simulink model "Thirtybussys1"  (R2021a)
settings: Solver=VariableStepAuto  StartTime=0.0  StopTime=4.0  RelTol=1e-3
libraries: spsFourierLib x60, spsThreePhaseSeriesRLCBranchLib x41, spsThreePhaseVIMeasurementLib x30, spsThreePhaseSeriesRLCLoadLib x21, spsThreePhaseSourceLib x6, spsThreePhaseTransformerTwoWindingsLib x6, spsThreePhaseFaultLib x2, spspowerguiLib x1
(part 2 of 2)

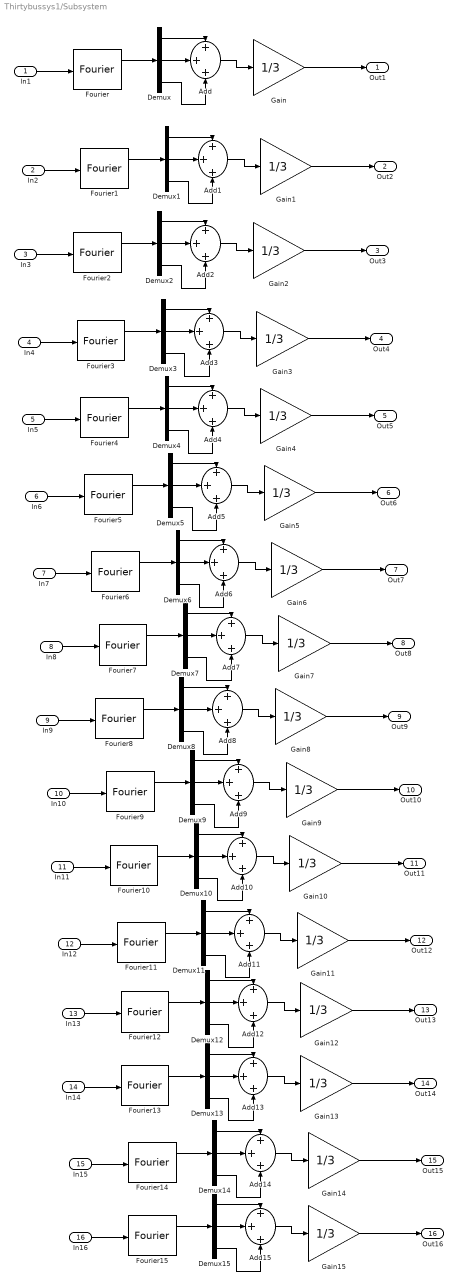
== system Thirtybussys1/Subsystem ==
  In1 : Inport
  In2 : Inport  Port=2
  In3 : Inport  Port=3
  In4 : Inport  Port=4
  In5 : Inport  Port=5
  In6 : Inport  Port=6
  In7 : Inport  Port=7
  In8 : Inport  Port=8
  In9 : Inport  Port=9
  In10 : Inport  Port=10
  In11 : Inport  Port=11
  In12 : Inport  Port=12
  In13 : Inport  Port=13
  In14 : Inport  Port=14
  In15 : Inport  Port=15
  In16 : Inport  Port=16
  Add{,1..15} (16 alike) : Sum  Inputs=+++
  Demux{,1..15} (16 alike) : Demux  Outputs=3
  Fourier{,1..15} (16 alike) : spsFourierLib/Fourier  Freq=60  n=1  InInit=[0, 0]  Ts=50e-6
      settings: SourceProductBaseCode=PS
  Gain{,1..15} (16 alike) : Gain  Gain=1/3
  Out1 : Outport
  Out2 : Outport  Port=2
  Out3 : Outport  Port=3
  Out4 : Outport  Port=4
  Out5 : Outport  Port=5
  Out6 : Outport  Port=6
  Out7 : Outport  Port=7
  Out8 : Outport  Port=8
  Out9 : Outport  Port=9
  Out10 : Outport  Port=10
  Out11 : Outport  Port=11
  Out12 : Outport  Port=12
  Out13 : Outport  Port=13
  Out14 : Outport  Port=14
  Out15 : Outport  Port=15
  Out16 : Outport  Port=16
  wires:
  In1/1 -> Fourier/1
  Add/1 -> Gain/1
  Gain/1 -> Out1/1
  Fourier/1 -> Demux/1
  Demux/1 -> Add/1
  Demux/2 -> Add/2
  Demux/3 -> Add/3
  Demux1/3 -> Add1/3
  Demux1/2 -> Add1/2
  In2/1 -> Fourier1/1
  Fourier1/1 -> Demux1/1
  Demux1/1 -> Add1/1
  Add1/1 -> Gain1/1
  Gain1/1 -> Out2/1
  Demux2/3 -> Add2/3
  Demux2/2 -> Add2/2
  In3/1 -> Fourier2/1
  Fourier2/1 -> Demux2/1
  Demux2/1 -> Add2/1
  Add2/1 -> Gain2/1
  Gain2/1 -> Out3/1
  Demux3/3 -> Add3/3
  Demux3/2 -> Add3/2
  In4/1 -> Fourier3/1
  Fourier3/1 -> Demux3/1
  Demux3/1 -> Add3/1
  Add3/1 -> Gain3/1
  Gain3/1 -> Out4/1
  Demux4/3 -> Add4/3
  Demux4/2 -> Add4/2
  In5/1 -> Fourier4/1
  Fourier4/1 -> Demux4/1
  Demux4/1 -> Add4/1
  Add4/1 -> Gain4/1
  Gain4/1 -> Out5/1
  Demux5/3 -> Add5/3
  Demux5/2 -> Add5/2
  In6/1 -> Fourier5/1
  Fourier5/1 -> Demux5/1
  Demux5/1 -> Add5/1
  Add5/1 -> Gain5/1
  Gain5/1 -> Out6/1
  Demux6/3 -> Add6/3
  Demux6/2 -> Add6/2
  In7/1 -> Fourier6/1
  Fourier6/1 -> Demux6/1
  Demux6/1 -> Add6/1
  Add6/1 -> Gain6/1
  Gain6/1 -> Out7/1
  Demux7/3 -> Add7/3
  Demux7/2 -> Add7/2
  In8/1 -> Fourier7/1
  Fourier7/1 -> Demux7/1
  Demux7/1 -> Add7/1
  Add7/1 -> Gain7/1
  Gain7/1 -> Out8/1
  Demux8/3 -> Add8/3
  Demux8/2 -> Add8/2
  In9/1 -> Fourier8/1
  Fourier8/1 -> Demux8/1
  Demux8/1 -> Add8/1
  Add8/1 -> Gain8/1
  Gain8/1 -> Out9/1
  Demux9/3 -> Add9/3
  Demux9/2 -> Add9/2
  In10/1 -> Fourier9/1
  Fourier9/1 -> Demux9/1
  Demux9/1 -> Add9/1
  Add9/1 -> Gain9/1
  Gain9/1 -> Out10/1
  Demux10/3 -> Add10/3
  Demux10/2 -> Add10/2
  In11/1 -> Fourier10/1
  Fourier10/1 -> Demux10/1
  Demux10/1 -> Add10/1
  Add10/1 -> Gain10/1
  Gain10/1 -> Out11/1
  Demux11/3 -> Add11/3
  Demux11/2 -> Add11/2
  In12/1 -> Fourier11/1
  Fourier11/1 -> Demux11/1
  Demux11/1 -> Add11/1
  Add11/1 -> Gain11/1
  Gain11/1 -> Out12/1
  Demux12/3 -> Add12/3
  Demux12/2 -> Add12/2
  In13/1 -> Fourier12/1
  Fourier12/1 -> Demux12/1
  Demux12/1 -> Add12/1
  Add12/1 -> Gain12/1
  Gain12/1 -> Out13/1
  Demux13/3 -> Add13/3
  Demux13/2 -> Add13/2
  In14/1 -> Fourier13/1
  Fourier13/1 -> Demux13/1
  Demux13/1 -> Add13/1
  Add13/1 -> Gain13/1
  Gain13/1 -> Out14/1
  Demux14/3 -> Add14/3
  Demux14/2 -> Add14/2
  In15/1 -> Fourier14/1
  Fourier14/1 -> Demux14/1
  Demux14/1 -> Add14/1
  Add14/1 -> Gain14/1
  Gain14/1 -> Out15/1
  Demux15/2 -> Add15/2
  Fourier15/1 -> Demux15/1
  Gain15/1 -> Out16/1
  In16/1 -> Fourier15/1
  Demux15/3 -> Add15/3
  Add15/1 -> Gain15/1
  Demux15/1 -> Add15/1

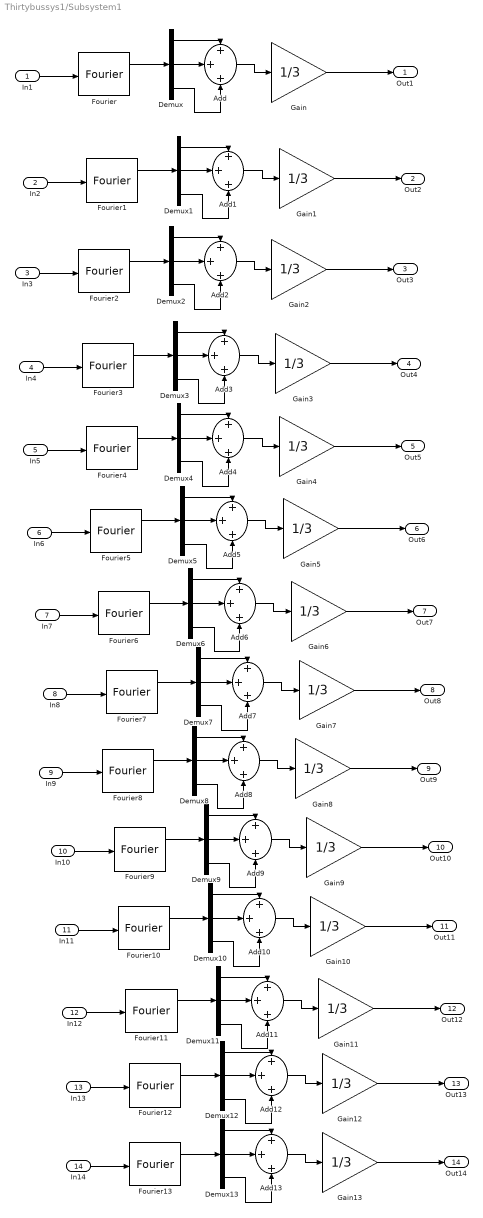
== system Thirtybussys1/Subsystem1 ==
  In1 : Inport
  In2 : Inport  Port=2
  In3 : Inport  Port=3
  In4 : Inport  Port=4
  In5 : Inport  Port=5
  In6 : Inport  Port=6
  In7 : Inport  Port=7
  In8 : Inport  Port=8
  In9 : Inport  Port=9
  In10 : Inport  Port=10
  In11 : Inport  Port=11
  In12 : Inport  Port=12
  In13 : Inport  Port=13
  In14 : Inport  Port=14
  Add{,1..13} (14 alike) : Sum  Inputs=+++
  Demux{,1..13} (14 alike) : Demux  Outputs=3
  Fourier{,1..13} (14 alike) : spsFourierLib/Fourier  Freq=60  n=1  InInit=[0, 0]  Ts=50e-6
      settings: SourceProductBaseCode=PS
  Gain{,1..13} (14 alike) : Gain  Gain=1/3
  Out1 : Outport
  Out2 : Outport  Port=2
  Out3 : Outport  Port=3
  Out4 : Outport  Port=4
  Out5 : Outport  Port=5
  Out6 : Outport  Port=6
  Out7 : Outport  Port=7
  Out8 : Outport  Port=8
  Out9 : Outport  Port=9
  Out10 : Outport  Port=10
  Out11 : Outport  Port=11
  Out12 : Outport  Port=12
  Out13 : Outport  Port=13
  Out14 : Outport  Port=14
  wires:
  In1/1 -> Fourier/1
  Add/1 -> Gain/1
  Gain/1 -> Out1/1
  Fourier/1 -> Demux/1
  Demux/1 -> Add/1
  Demux/2 -> Add/2
  Demux/3 -> Add/3
  Demux1/3 -> Add1/3
  Demux1/2 -> Add1/2
  In2/1 -> Fourier1/1
  Fourier1/1 -> Demux1/1
  Demux1/1 -> Add1/1
  Add1/1 -> Gain1/1
  Gain1/1 -> Out2/1
  Demux2/3 -> Add2/3
  Demux2/2 -> Add2/2
  In3/1 -> Fourier2/1
  Fourier2/1 -> Demux2/1
  Demux2/1 -> Add2/1
  Add2/1 -> Gain2/1
  Gain2/1 -> Out3/1
  Demux3/3 -> Add3/3
  Demux3/2 -> Add3/2
  In4/1 -> Fourier3/1
  Fourier3/1 -> Demux3/1
  Demux3/1 -> Add3/1
  Add3/1 -> Gain3/1
  Gain3/1 -> Out4/1
  Demux4/3 -> Add4/3
  Demux4/2 -> Add4/2
  In5/1 -> Fourier4/1
  Fourier4/1 -> Demux4/1
  Demux4/1 -> Add4/1
  Add4/1 -> Gain4/1
  Gain4/1 -> Out5/1
  Demux5/3 -> Add5/3
  Demux5/2 -> Add5/2
  In6/1 -> Fourier5/1
  Fourier5/1 -> Demux5/1
  Demux5/1 -> Add5/1
  Add5/1 -> Gain5/1
  Gain5/1 -> Out6/1
  Demux6/3 -> Add6/3
  Demux6/2 -> Add6/2
  In7/1 -> Fourier6/1
  Fourier6/1 -> Demux6/1
  Demux6/1 -> Add6/1
  Add6/1 -> Gain6/1
  Gain6/1 -> Out7/1
  Demux7/3 -> Add7/3
  Demux7/2 -> Add7/2
  In8/1 -> Fourier7/1
  Fourier7/1 -> Demux7/1
  Demux7/1 -> Add7/1
  Add7/1 -> Gain7/1
  Gain7/1 -> Out8/1
  Demux8/3 -> Add8/3
  Demux8/2 -> Add8/2
  In9/1 -> Fourier8/1
  Fourier8/1 -> Demux8/1
  Demux8/1 -> Add8/1
  Add8/1 -> Gain8/1
  Gain8/1 -> Out9/1
  Demux9/3 -> Add9/3
  Demux9/2 -> Add9/2
  In10/1 -> Fourier9/1
  Fourier9/1 -> Demux9/1
  Demux9/1 -> Add9/1
  Add9/1 -> Gain9/1
  Gain9/1 -> Out10/1
  Demux10/3 -> Add10/3
  Demux10/2 -> Add10/2
  In11/1 -> Fourier10/1
  Fourier10/1 -> Demux10/1
  Demux10/1 -> Add10/1
  Add10/1 -> Gain10/1
  Gain10/1 -> Out11/1
  Demux11/3 -> Add11/3
  Demux11/2 -> Add11/2
  In12/1 -> Fourier11/1
  Fourier11/1 -> Demux11/1
  Demux11/1 -> Add11/1
  Add11/1 -> Gain11/1
  Gain11/1 -> Out12/1
  Demux12/3 -> Add12/3
  Demux12/2 -> Add12/2
  In13/1 -> Fourier12/1
  Fourier12/1 -> Demux12/1
  Demux12/1 -> Add12/1
  Add12/1 -> Gain12/1
  Gain12/1 -> Out13/1
  Demux13/3 -> Add13/3
  Demux13/2 -> Add13/2
  In14/1 -> Fourier13/1
  Fourier13/1 -> Demux13/1
  Demux13/1 -> Add13/1
  Add13/1 -> Gain13/1
  Gain13/1 -> Out14/1

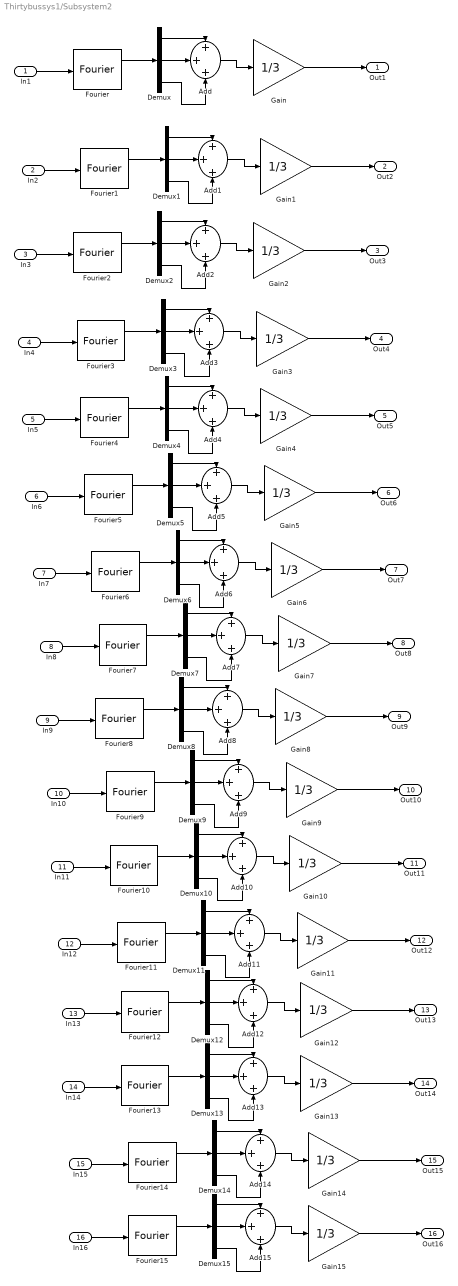
== system Thirtybussys1/Subsystem2 ==
  In1 : Inport
  In2 : Inport  Port=2
  In3 : Inport  Port=3
  In4 : Inport  Port=4
  In5 : Inport  Port=5
  In6 : Inport  Port=6
  In7 : Inport  Port=7
  In8 : Inport  Port=8
  In9 : Inport  Port=9
  In10 : Inport  Port=10
  In11 : Inport  Port=11
  In12 : Inport  Port=12
  In13 : Inport  Port=13
  In14 : Inport  Port=14
  In15 : Inport  Port=15
  In16 : Inport  Port=16
  Add{,1..15} (16 alike) : Sum  Inputs=+++
  Demux{,1..15} (16 alike) : Demux  Outputs=3
  Fourier{,1..15} (16 alike) : spsFourierLib/Fourier  Freq=60  n=1  InInit=[0, 0]  Ts=50e-6
      settings: SourceProductBaseCode=PS
  Gain{,1..15} (16 alike) : Gain  Gain=1/3
  Out1 : Outport
  Out2 : Outport  Port=2
  Out3 : Outport  Port=3
  Out4 : Outport  Port=4
  Out5 : Outport  Port=5
  Out6 : Outport  Port=6
  Out7 : Outport  Port=7
  Out8 : Outport  Port=8
  Out9 : Outport  Port=9
  Out10 : Outport  Port=10
  Out11 : Outport  Port=11
  Out12 : Outport  Port=12
  Out13 : Outport  Port=13
  Out14 : Outport  Port=14
  Out15 : Outport  Port=15
  Out16 : Outport  Port=16
  wires:
  In1/1 -> Fourier/1
  Add/1 -> Gain/1
  Gain/1 -> Out1/1
  Fourier/1 -> Demux/1
  Demux/1 -> Add/1
  Demux/2 -> Add/2
  Demux/3 -> Add/3
  Demux1/3 -> Add1/3
  Demux1/2 -> Add1/2
  In2/1 -> Fourier1/1
  Fourier1/1 -> Demux1/1
  Demux1/1 -> Add1/1
  Add1/1 -> Gain1/1
  Gain1/1 -> Out2/1
  Demux2/3 -> Add2/3
  Demux2/2 -> Add2/2
  In3/1 -> Fourier2/1
  Fourier2/1 -> Demux2/1
  Demux2/1 -> Add2/1
  Add2/1 -> Gain2/1
  Gain2/1 -> Out3/1
  Demux3/3 -> Add3/3
  Demux3/2 -> Add3/2
  In4/1 -> Fourier3/1
  Fourier3/1 -> Demux3/1
  Demux3/1 -> Add3/1
  Add3/1 -> Gain3/1
  Gain3/1 -> Out4/1
  Demux4/3 -> Add4/3
  Demux4/2 -> Add4/2
  In5/1 -> Fourier4/1
  Fourier4/1 -> Demux4/1
  Demux4/1 -> Add4/1
  Add4/1 -> Gain4/1
  Gain4/1 -> Out5/1
  Demux5/3 -> Add5/3
  Demux5/2 -> Add5/2
  In6/1 -> Fourier5/1
  Fourier5/1 -> Demux5/1
  Demux5/1 -> Add5/1
  Add5/1 -> Gain5/1
  Gain5/1 -> Out6/1
  Demux6/3 -> Add6/3
  Demux6/2 -> Add6/2
  In7/1 -> Fourier6/1
  Fourier6/1 -> Demux6/1
  Demux6/1 -> Add6/1
  Add6/1 -> Gain6/1
  Gain6/1 -> Out7/1
  Demux7/3 -> Add7/3
  Demux7/2 -> Add7/2
  In8/1 -> Fourier7/1
  Fourier7/1 -> Demux7/1
  Demux7/1 -> Add7/1
  Add7/1 -> Gain7/1
  Gain7/1 -> Out8/1
  Demux8/3 -> Add8/3
  Demux8/2 -> Add8/2
  In9/1 -> Fourier8/1
  Fourier8/1 -> Demux8/1
  Demux8/1 -> Add8/1
  Add8/1 -> Gain8/1
  Gain8/1 -> Out9/1
  Demux9/3 -> Add9/3
  Demux9/2 -> Add9/2
  In10/1 -> Fourier9/1
  Fourier9/1 -> Demux9/1
  Demux9/1 -> Add9/1
  Add9/1 -> Gain9/1
  Gain9/1 -> Out10/1
  Demux10/3 -> Add10/3
  Demux10/2 -> Add10/2
  In11/1 -> Fourier10/1
  Fourier10/1 -> Demux10/1
  Demux10/1 -> Add10/1
  Add10/1 -> Gain10/1
  Gain10/1 -> Out11/1
  Demux11/3 -> Add11/3
  Demux11/2 -> Add11/2
  In12/1 -> Fourier11/1
  Fourier11/1 -> Demux11/1
  Demux11/1 -> Add11/1
  Add11/1 -> Gain11/1
  Gain11/1 -> Out12/1
  Demux12/3 -> Add12/3
  Demux12/2 -> Add12/2
  In13/1 -> Fourier12/1
  Fourier12/1 -> Demux12/1
  Demux12/1 -> Add12/1
  Add12/1 -> Gain12/1
  Gain12/1 -> Out13/1
  Demux13/3 -> Add13/3
  Demux13/2 -> Add13/2
  In14/1 -> Fourier13/1
  Fourier13/1 -> Demux13/1
  Demux13/1 -> Add13/1
  Add13/1 -> Gain13/1
  Gain13/1 -> Out14/1
  Demux14/3 -> Add14/3
  Demux14/2 -> Add14/2
  In15/1 -> Fourier14/1
  Fourier14/1 -> Demux14/1
  Demux14/1 -> Add14/1
  Add14/1 -> Gain14/1
  Gain14/1 -> Out15/1
  Demux15/2 -> Add15/2
  Fourier15/1 -> Demux15/1
  Gain15/1 -> Out16/1
  In16/1 -> Fourier15/1
  Demux15/3 -> Add15/3
  Add15/1 -> Gain15/1
  Demux15/1 -> Add15/1

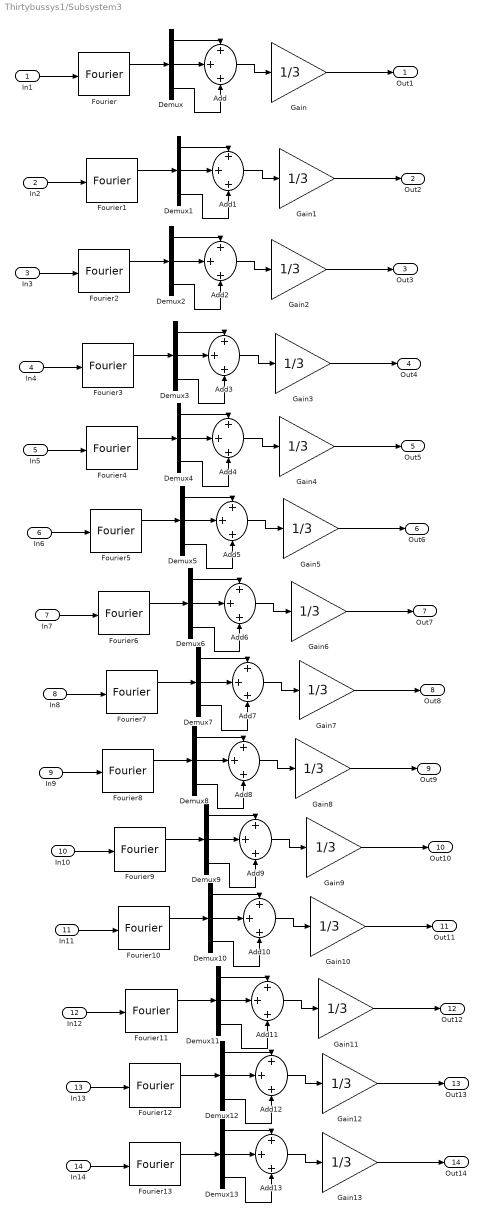
== system Thirtybussys1/Subsystem3 ==
  In1 : Inport
  In2 : Inport  Port=2
  In3 : Inport  Port=3
  In4 : Inport  Port=4
  In5 : Inport  Port=5
  In6 : Inport  Port=6
  In7 : Inport  Port=7
  In8 : Inport  Port=8
  In9 : Inport  Port=9
  In10 : Inport  Port=10
  In11 : Inport  Port=11
  In12 : Inport  Port=12
  In13 : Inport  Port=13
  In14 : Inport  Port=14
  Add{,1..13} (14 alike) : Sum  Inputs=+++
  Demux{,1..13} (14 alike) : Demux  Outputs=3
  Fourier{,1..13} (14 alike) : spsFourierLib/Fourier  Freq=60  n=1  InInit=[0, 0]  Ts=50e-6
      settings: SourceProductBaseCode=PS
  Gain{,1..13} (14 alike) : Gain  Gain=1/3
  Out1 : Outport
  Out2 : Outport  Port=2
  Out3 : Outport  Port=3
  Out4 : Outport  Port=4
  Out5 : Outport  Port=5
  Out6 : Outport  Port=6
  Out7 : Outport  Port=7
  Out8 : Outport  Port=8
  Out9 : Outport  Port=9
  Out10 : Outport  Port=10
  Out11 : Outport  Port=11
  Out12 : Outport  Port=12
  Out13 : Outport  Port=13
  Out14 : Outport  Port=14
  wires:
  In1/1 -> Fourier/1
  Add/1 -> Gain/1
  Gain/1 -> Out1/1
  Fourier/1 -> Demux/1
  Demux/1 -> Add/1
  Demux/2 -> Add/2
  Demux/3 -> Add/3
  Demux1/3 -> Add1/3
  Demux1/2 -> Add1/2
  In2/1 -> Fourier1/1
  Fourier1/1 -> Demux1/1
  Demux1/1 -> Add1/1
  Add1/1 -> Gain1/1
  Gain1/1 -> Out2/1
  Demux2/3 -> Add2/3
  Demux2/2 -> Add2/2
  In3/1 -> Fourier2/1
  Fourier2/1 -> Demux2/1
  Demux2/1 -> Add2/1
  Add2/1 -> Gain2/1
  Gain2/1 -> Out3/1
  Demux3/3 -> Add3/3
  Demux3/2 -> Add3/2
  In4/1 -> Fourier3/1
  Fourier3/1 -> Demux3/1
  Demux3/1 -> Add3/1
  Add3/1 -> Gain3/1
  Gain3/1 -> Out4/1
  Demux4/3 -> Add4/3
  Demux4/2 -> Add4/2
  In5/1 -> Fourier4/1
  Fourier4/1 -> Demux4/1
  Demux4/1 -> Add4/1
  Add4/1 -> Gain4/1
  Gain4/1 -> Out5/1
  Demux5/3 -> Add5/3
  Demux5/2 -> Add5/2
  In6/1 -> Fourier5/1
  Fourier5/1 -> Demux5/1
  Demux5/1 -> Add5/1
  Add5/1 -> Gain5/1
  Gain5/1 -> Out6/1
  Demux6/3 -> Add6/3
  Demux6/2 -> Add6/2
  In7/1 -> Fourier6/1
  Fourier6/1 -> Demux6/1
  Demux6/1 -> Add6/1
  Add6/1 -> Gain6/1
  Gain6/1 -> Out7/1
  Demux7/3 -> Add7/3
  Demux7/2 -> Add7/2
  In8/1 -> Fourier7/1
  Fourier7/1 -> Demux7/1
  Demux7/1 -> Add7/1
  Add7/1 -> Gain7/1
  Gain7/1 -> Out8/1
  Demux8/3 -> Add8/3
  Demux8/2 -> Add8/2
  In9/1 -> Fourier8/1
  Fourier8/1 -> Demux8/1
  Demux8/1 -> Add8/1
  Add8/1 -> Gain8/1
  Gain8/1 -> Out9/1
  Demux9/3 -> Add9/3
  Demux9/2 -> Add9/2
  In10/1 -> Fourier9/1
  Fourier9/1 -> Demux9/1
  Demux9/1 -> Add9/1
  Add9/1 -> Gain9/1
  Gain9/1 -> Out10/1
  Demux10/3 -> Add10/3
  Demux10/2 -> Add10/2
  In11/1 -> Fourier10/1
  Fourier10/1 -> Demux10/1
  Demux10/1 -> Add10/1
  Add10/1 -> Gain10/1
  Gain10/1 -> Out11/1
  Demux11/3 -> Add11/3
  Demux11/2 -> Add11/2
  In12/1 -> Fourier11/1
  Fourier11/1 -> Demux11/1
  Demux11/1 -> Add11/1
  Add11/1 -> Gain11/1
  Gain11/1 -> Out12/1
  Demux12/3 -> Add12/3
  Demux12/2 -> Add12/2
  In13/1 -> Fourier12/1
  Fourier12/1 -> Demux12/1
  Demux12/1 -> Add12/1
  Add12/1 -> Gain12/1
  Gain12/1 -> Out13/1
  Demux13/3 -> Add13/3
  Demux13/2 -> Add13/2
  In14/1 -> Fourier13/1
  Fourier13/1 -> Demux13/1
  Demux13/1 -> Add13/1
  Add13/1 -> Gain13/1
  Gain13/1 -> Out14/1
